simulink model "baseon_BD_iter"  (R2017b)
settings: Solver=VariableStepAuto  StartTime=0.0  StopTime=15  RelTol=1e-3
PreLoadFcn:
  | init.m;
libraries: simulink x1
settings Model: Creator=Administrator  LastModifiedBy=Administrator
settings SolverCC: ZeroCrossAlgorithm=Adaptive  AlgebraicLoopSolver=LineSearch
settings DebuggingCC: MaxConsecutiveZCsMsg=none

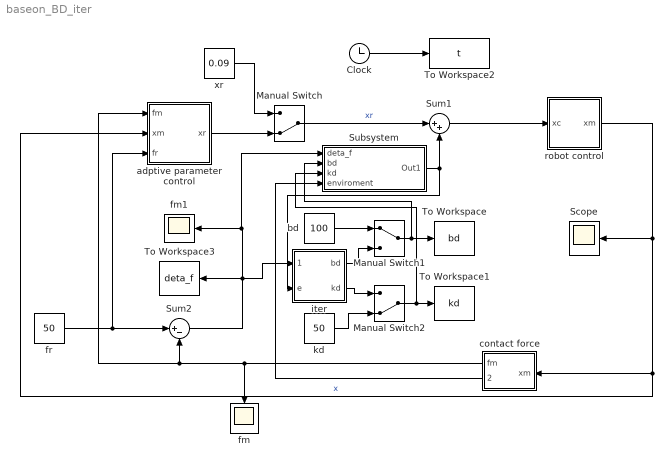
== system baseon_BD_iter ==
  Clock : Clock
  Manual Switch : ManualSwitch  CurrentSetting=0
  Manual Switch1 : ManualSwitch
  Manual Switch2 : ManualSwitch  CurrentSetting=0
  Scope : Scope
  Subsystem : Subsystem
  Sum1 : Sum  Inputs=|++
  Sum2 : Sum  Inputs=|+-
  To Workspace : ToWorkspace  VariableName=bd  SampleTime=-1
      settings: Save2DSignal=2-D array (concatenate along first dimension)
  To Workspace1 : ToWorkspace  VariableName=kd  SampleTime=-1
      settings: Save2DSignal=2-D array (concatenate along first dimension)
  To Workspace2 : ToWorkspace  VariableName=t  SampleTime=-1
  To Workspace3 : ToWorkspace  VariableName=deta_f  SampleTime=-1
      settings: Save2DSignal=2-D array (concatenate along first dimension)
  adptive parameter control : Subsystem
  bd : Constant  Value=100
  contact force : Subsystem
  fm : Scope
  fm1 : Scope
  fr : Constant  Value=50
  iter : Subsystem
  kd : Constant  Value=50
  robot control : Subsystem
  xr : Constant  Value=0.09
  wires:
  adptive parameter control/1(xr) -> Manual Switch/2
  xr/1 -> Manual Switch/1
  fr/1 -> adptive parameter control/3(fr), Sum2/1
  Sum1/1 -> robot control/1(xc)
  Manual Switch1/1 -> Subsystem/2(bd), To Workspace/1
  robot control/1("xm ") -> adptive parameter control/2(xm), contact force/1(xm), Scope/1  "x"
  contact force/1("fm ") -> fm/1, Sum2/2, adptive parameter control/1(fm)
  Sum2/1 -> iter/1(deta_f), To Workspace3/1, Subsystem/1(deta_f), fm1/1
  Clock/1 -> To Workspace2/1
  iter/1("bd ") -> Manual Switch1/2
  bd/1 -> Manual Switch1/1
  iter/2(kd) -> Manual Switch2/1
  Manual Switch2/1 -> Subsystem/3(kd), To Workspace1/1
  kd/1 -> Manual Switch2/2
  Subsystem/1(Out1) -> iter/2(e), Sum1/2
  Manual Switch/1 -> Sum1/1  "xr"
  contact force/2(enviroment) -> Subsystem/4(enviroment)

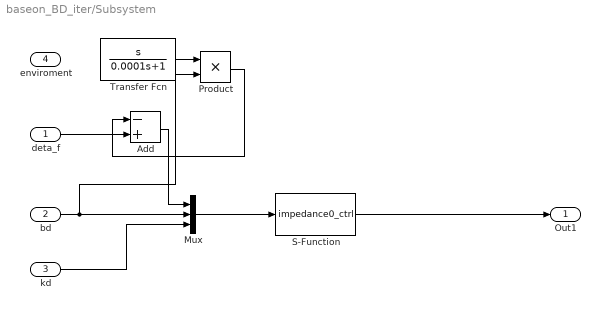
== system baseon_BD_iter/Subsystem ==
  deta_f : Inport
  bd : Inport  Port=2
  kd : Inport  Port=3
  enviroment : Inport  Port=4
  Add : Sum  Inputs=-+
  Mux : Mux  Inputs=3
  Product : Product
  S-Function : S-Function  FunctionName=impedance0_ctrl  SFunctionDeploymentMode=off  EnableBusSupport=off
  Transfer Fcn : TransferFcn  Numerator=[1 0]  Denominator=[0.0001 1]
  Out1 : Outport
  wires:
  bd/1 -> Product/2, Mux/2
  kd/1 -> Mux/3
  Mux/1 -> S-Function/1
  S-Function/1 -> Out1/1
  Transfer Fcn/1 -> Product/1
  deta_f/1 -> Add/2
  Add/1 -> Mux/1
  Product/1 -> Add/1

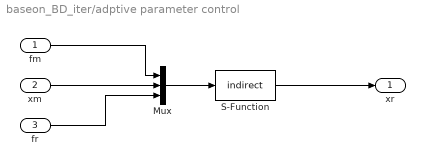
== system baseon_BD_iter/adptive parameter control ==
  fm : Inport
  xm : Inport  Port=2
  fr : Inport  Port=3
  Mux : Mux  Inputs=3
  S-Function : S-Function  FunctionName=indirect  SFunctionDeploymentMode=off  EnableBusSupport=off
  xr : Outport
  wires:
  fm/1 -> Mux/1
  xm/1 -> Mux/2
  Mux/1 -> S-Function/1
  S-Function/1 -> xr/1
  fr/1 -> Mux/3

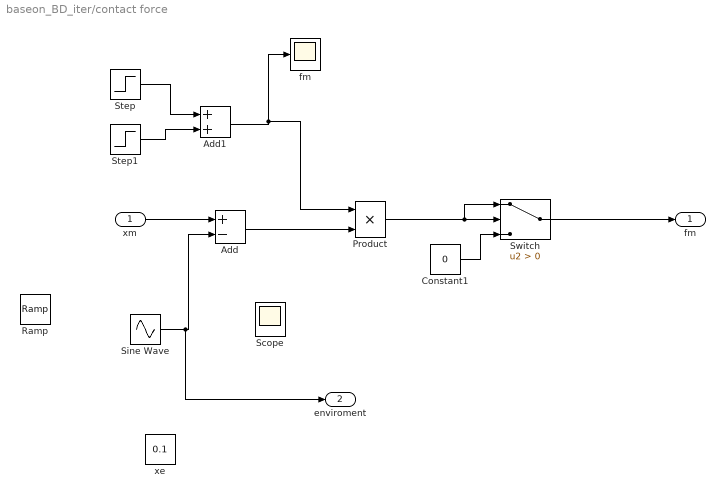
== system baseon_BD_iter/contact force ==
  xm : Inport
  Add : Sum  Inputs=+-
  Add1 : Sum
  Constant1 : Constant  Value=0
  Product : Product
  Ramp : simulink/Sources/Ramp  slope=0.1  start=0  X0=0
  Scope : Scope
  Sine Wave : Sin  Amplitude=0.3  Bias=0.1  SampleTime=0
  Step : Step  Time=100  Before=1500  After=2500  SampleTime=0
  Step1 : Step  Time=100  After=1500  SampleTime=0
  Switch : Switch  Criteria=u2 > Threshold
  fm : Scope
  xe : Constant  Value=0.1
  "fm " : Outport
  enviroment : Outport  Port=2
  wires:
  xm/1 -> Add/1
  Add/1 -> Product/2
  Constant1/1 -> Switch/3
  Step/1 -> Add1/1
  Step1/1 -> Add1/2
  Add1/1 -> Product/1, fm/1
  Product/1 -> Switch/1, Switch/2
  Switch/1 -> "fm "/1
  Sine Wave/1 -> enviroment/1, Add/2

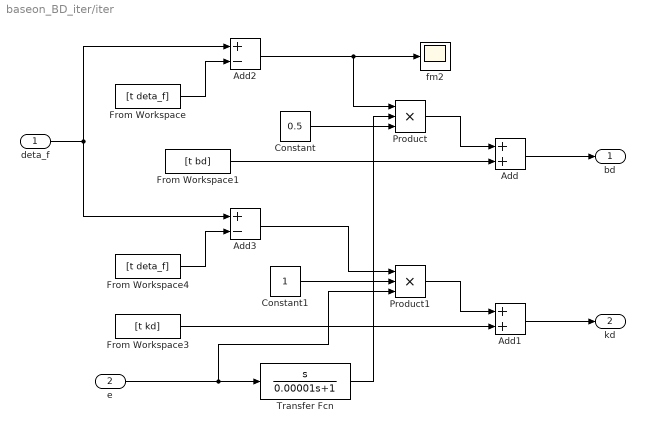
== system baseon_BD_iter/iter ==
  deta_f : Inport
  e : Inport  Port=2
  Add : Sum
  Add1 : Sum
  Add2 : Sum  Inputs=+-
  Add3 : Sum  Inputs=+-
  Constant : Constant  Value=0.5
  Constant1 : Constant
  From Workspace : FromWorkspace  VariableName=[t deta_f]  SampleTime=0
  From Workspace1 : FromWorkspace  VariableName=[t bd]  SampleTime=0
  From Workspace3 : FromWorkspace  VariableName=[t kd]  SampleTime=0
  From Workspace4 : FromWorkspace  VariableName=[t deta_f]  SampleTime=0
  Product : Product  Inputs=3
  Product1 : Product  Inputs=3
  Transfer Fcn : TransferFcn  Numerator=[1 0]  Denominator=[0.00001 1]
  fm2 : Scope
  "bd " : Outport
  kd : Outport  Port=2
  wires:
  Constant/1 -> Product/3
  Product/1 -> Add/1
  Add/1 -> "bd "/1
  From Workspace1/1 -> Add/2
  Product1/1 -> Add1/1
  Constant1/1 -> Product1/2
  From Workspace3/1 -> Add1/2
  Add1/1 -> kd/1
  deta_f/1 -> Add3/1, Add2/1
  From Workspace/1 -> Add2/2
  Add2/1 -> fm2/1, Product/1
  From Workspace4/1 -> Add3/2
  Add3/1 -> Product1/1
  e/1 -> Product1/3, Transfer Fcn/1
  Transfer Fcn/1 -> Product/2

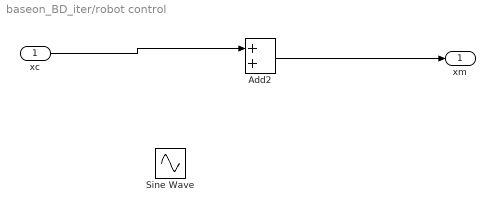
== system baseon_BD_iter/robot control ==
  xc : Inport
  Add2 : Sum
  Sine Wave : Sin  Amplitude=0.02  Bias=0.02  Frequency=0.22  SampleTime=0
  "xm " : Outport
  wires:
  xc/1 -> Add2/1
  Add2/1 -> "xm "/1
